simulink model "Backstepping_Quadrator_Attitude"  (R2018a)
settings: Solver=ode4  StartTime=0.0  StopTime=12  FixedStep=1e-4  MaxStep=1e-3  MinStep=1e-4  RelTol=1e-3
libraries: simulink x8, powerlib_meascontrol x1
settings Model: Creator=oussa  LastModifiedBy=oussa

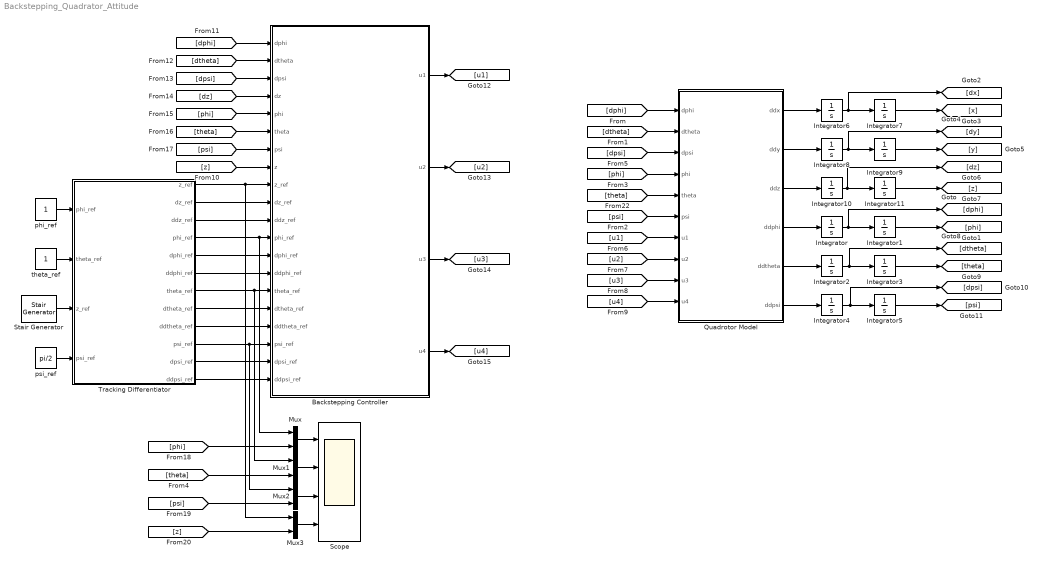
== system Backstepping_Quadrator_Attitude ==
  Backstepping Controller : MATLAB Function  TreatAsAtomicUnit=on
  Integrator : Integrator  InitialCondition=0.001
  Integrator{1..11} (11 alike) : Integrator
  Mux{,1..3} (4 alike) : Mux  Inputs=2
  Quadrotor Model : MATLAB Function  TreatAsAtomicUnit=on
  Scope : Scope  NumInputPorts=4
  Stair Generator : powerlib_meascontrol/Pulse & Signal Generators/Stair Generator  t=[0, 1,3, 5, 8.5,10,12]  e=[0,5,2,9,15,0,0]  Ts=0
      settings: SourceProductName=Simscape Power Systems
  Tracking Differentiator : Subsystem
  phi_ref : Constant
  psi_ref : Constant  Value=pi/2
  theta_ref : Constant
  wires:
  Quadrotor Model/4(ddphi) -> Integrator/1
  Quadrotor Model/5(ddtheta) -> Integrator2/1
  Quadrotor Model/6(ddpsi) -> Integrator4/1
  Integrator10/1 -> [dz], Integrator11/1
  Integrator8/1 -> [dy], Integrator9/1
  Quadrotor Model/1(ddx) -> Integrator6/1
  Quadrotor Model/3(ddz) -> Integrator10/1
  Quadrotor Model/2(ddy) -> Integrator8/1
  Integrator4/1 -> [dpsi], Integrator5/1
  Integrator2/1 -> Integrator3/1, [dtheta]
  Integrator/1 -> Integrator1/1, [dphi]
  Integrator1/1 -> [phi]
  Integrator7/1 -> [x]
  Integrator6/1 -> [dx], Integrator7/1
  Integrator9/1 -> [y]
  Integrator11/1 -> [z]
  Integrator3/1 -> [theta]
  Integrator5/1 -> [psi]
  [dphi] -> Quadrotor Model/1(dphi)
  [dtheta] -> Quadrotor Model/2(dtheta)
  [phi] -> Quadrotor Model/4(phi)
  [theta] -> Quadrotor Model/5(theta)
  [dpsi] -> Quadrotor Model/3(dpsi)
  [psi] -> Quadrotor Model/6(psi)
  [u1] -> Quadrotor Model/7(u1)
  [u2] -> Quadrotor Model/8(u2)
  [u3] -> Quadrotor Model/9(u3)
  [u4] -> Quadrotor Model/10(u4)
  Mux/1 -> Scope/1
  Mux1/1 -> Scope/2
  [psi] -> Mux2/2
  [z] -> Mux3/2
  Mux2/1 -> Scope/3
  Mux3/1 -> Scope/4
  Backstepping Controller/2(u2) -> [u2]
  [z] -> Backstepping Controller/8(z)
  [psi] -> Backstepping Controller/7(psi)
  [theta] -> Backstepping Controller/6(theta)
  [phi] -> Backstepping Controller/5(phi)
  Backstepping Controller/3(u3) -> [u3]
  Backstepping Controller/4(u4) -> [u4]
  [dphi] -> Backstepping Controller/1(dphi)
  [dtheta] -> Backstepping Controller/2(dtheta)
  [dz] -> Backstepping Controller/4(dz)
  [dpsi] -> Backstepping Controller/3(dpsi)
  Tracking Differentiator/1("z_ref ") -> Mux3/1, Backstepping Controller/9(z_ref)
  Tracking Differentiator/2(dz_ref) -> Backstepping Controller/10(dz_ref)
  Tracking Differentiator/3(ddz_ref) -> Backstepping Controller/11(ddz_ref)
  Tracking Differentiator/4("phi_ref ") -> Mux/1, Backstepping Controller/12(phi_ref)
  Tracking Differentiator/5(dphi_ref) -> Backstepping Controller/13(dphi_ref)
  Tracking Differentiator/6(ddphi_ref) -> Backstepping Controller/14(ddphi_ref)
  Tracking Differentiator/7("theta_ref ") -> Mux1/1, Backstepping Controller/15(theta_ref)
  Tracking Differentiator/8("dtheta_ref ") -> Backstepping Controller/16(dtheta_ref)
  Tracking Differentiator/9(ddtheta_ref) -> Backstepping Controller/17(ddtheta_ref)
  Tracking Differentiator/11(dpsi_ref) -> Backstepping Controller/19(dpsi_ref)
  Tracking Differentiator/12(ddpsi_ref) -> Backstepping Controller/20(ddpsi_ref)
  phi_ref/1 -> Tracking Differentiator/1(phi_ref)
  theta_ref/1 -> Tracking Differentiator/2(theta_ref)
  [theta] -> Mux1/2
  [phi] -> Mux/2
  Tracking Differentiator/10("psi_ref ") -> Mux2/1, Backstepping Controller/18(psi_ref)
  psi_ref/1 -> Tracking Differentiator/4(psi_ref)
  Stair Generator/1 -> Tracking Differentiator/3(z_ref)
  Backstepping Controller/1(u1) -> [u1]

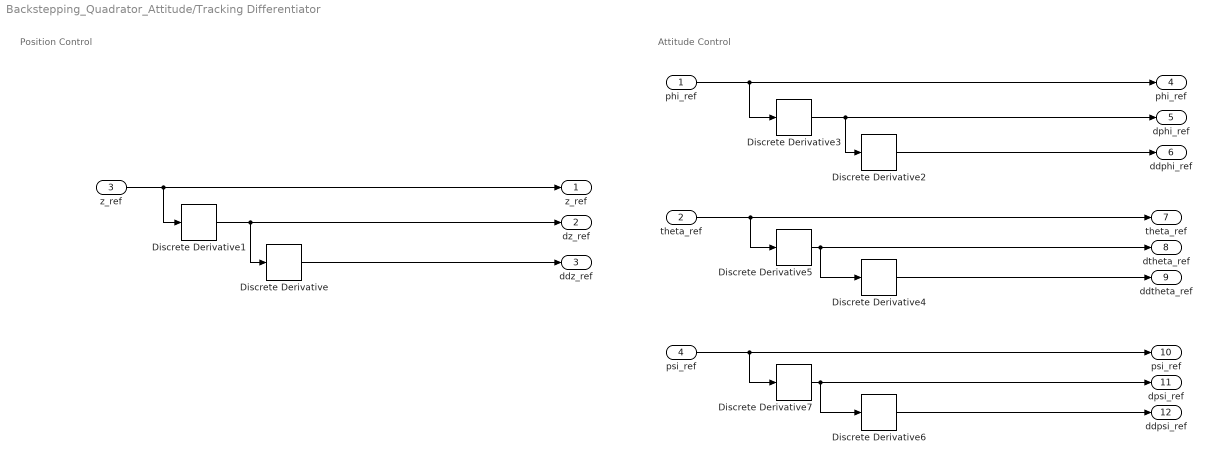
== system Backstepping_Quadrator_Attitude/Tracking Differentiator ==
  note: Attitude Control
  note: Position Control
  phi_ref : Inport
  theta_ref : Inport  Port=2
  z_ref : Inport  Port=3
  psi_ref : Inport  Port=4
  Discrete Derivative{,1..7} (8 alike) : simulink/Discrete/Discrete Derivative  gainval=eps  ICPrevScaledInput=0.0  OutMin=[]  OutMax=[]  OutDataType=fixdt(1, 16)  OutScaling=2^-10  DoSatur=off
  "z_ref " : Outport
  dz_ref : Outport  Port=2
  ddz_ref : Outport  Port=3
  "phi_ref " : Outport  Port=4
  dphi_ref : Outport  Port=5
  ddphi_ref : Outport  Port=6
  "theta_ref " : Outport  Port=7
  "dtheta_ref " : Outport  Port=8
  ddtheta_ref : Outport  Port=9
  "psi_ref " : Outport  Port=10
  dpsi_ref : Outport  Port=11
  ddpsi_ref : Outport  Port=12
  wires:
  Discrete Derivative/1 -> ddz_ref/1
  Discrete Derivative4/1 -> ddtheta_ref/1
  Discrete Derivative1/1 -> Discrete Derivative/1, dz_ref/1
  Discrete Derivative3/1 -> dphi_ref/1, Discrete Derivative2/1
  Discrete Derivative5/1 -> "dtheta_ref "/1, Discrete Derivative4/1
  phi_ref/1 -> "phi_ref "/1, Discrete Derivative3/1
  Discrete Derivative2/1 -> ddphi_ref/1
  theta_ref/1 -> Discrete Derivative5/1, "theta_ref "/1
  psi_ref/1 -> Discrete Derivative7/1, "psi_ref "/1
  Discrete Derivative7/1 -> dpsi_ref/1, Discrete Derivative6/1
  Discrete Derivative6/1 -> ddpsi_ref/1
  z_ref/1 -> Discrete Derivative1/1, "z_ref "/1

== matlab function Backstepping_Quadrator_Attitude/Backstepping Controller ==
  data: dphi input; dtheta input; dpsi input; dz input; phi input; theta input; psi input; z input; z_ref input; dz_ref input; ddz_ref input; phi_ref input; dphi_ref input; ddphi_ref input; theta_ref input; dtheta_ref input; u1 output; u2 output; u3 output; u4 output; ddtheta_ref input; psi_ref input; dpsi_ref input; ddpsi_ref input
function [u1,u2,u3,u4] = Backstepping_Controller(dphi,dtheta,dpsi,dz,phi,theta,psi,z,z_ref,dz_ref,ddz_ref,phi_ref,dphi_ref,ddphi_ref,theta_ref,dtheta_ref,ddtheta_ref,psi_ref,dpsi_ref,ddpsi_ref)
m = 2;
Ix = 1.25;
Iy = 1.25;
Iz = 2.2;
Ir = 1;
g = 9.8;
w = 10;

a1 = (Iy-Iz)/Ix; a2 = -Ir/Ix*w; b1 = 1/Ix;
a3 = (Iz-Ix)/Iy; a4 = Ir/Iy*w; b2 = 1/Iy;
a5= (Ix-Iy)/Iz; b3 = 1/Iz;

k1 = 20;
k2 = k1;
k3 = k1;
k4 = k1;
k5 = k1;
k6 = k1;
k7 = k1;
k8 = k1;

e1 = phi_ref-phi;
e2 = dphi-k1*e1-dphi_ref;
u2 = 1/b1*(-k2*e2+e1+ddphi_ref-k1*(e2+k1*e1)-a1*dtheta*dpsi-a2*dtheta*w);

e3 = theta_ref-theta;
e4 = dtheta-dtheta_ref-k3*e3;
u3 = 1/b2*(-k4*e4+e3-a3*dphi*dpsi-a4*w*dphi+ddtheta_ref-k3*(e4+k3*e3));

e5 = psi_ref-psi;
e6 = dpsi-dpsi_ref-k5*e5;
u4 = 1/b3*(-k6*e6+e5-a5*dphi*dtheta+ddpsi_ref-k5*(e6+k5*e5));

e7 = z_ref-z;
e8 = dz-dz_ref-k7*e7;
u1 = m/(cos(phi)*cos(theta))*(-k8*e8+e7+g-k7*(e8+k7*e7)+ddz_ref);

end

== matlab function Backstepping_Quadrator_Attitude/Quadrotor Model ==
  data: ddx output size=1; dphi input size=1; dtheta input size=1; dpsi input size=1; phi input size=1; theta input size=1; psi input size=1; u1 input size=1; u2 input size=1; u3 input size=1; u4 input size=1; ddy output size=1; ddz output size=1; ddphi output size=1; ddtheta output size=1; ddpsi output size=1
function [ddx,ddy,ddz,ddphi,ddtheta,ddpsi] = Quadrotor(dphi,dtheta,dpsi,phi,theta,psi,u1,u2,u3,u4)
m = 2;
Ix = 1.25;
Iy = 1.25;
Iz = 2.2;
Ir = 1;
g = 9.8;
w = 10;
a1 = (Iy-Iz)/Ix; a2 = -Ir/Ix*w; a3 = 1/Ix;
b1 = (Iz-Ix)/Iy; b2 = Ir/Iy*w; b3 = 1/Iy;
c1= (Ix-Iy)/Iz; c2 = 1/Iz;

ddx = (cos(phi)*sin(theta)*cos(psi)+sin(phi)*sin(psi))*u1/m;
ddy = (cos(phi)*sin(theta)*sin(psi)-sin(phi)*cos(psi))*u1/m;
ddz = -g+(cos(theta)*cos(phi))*u1/m;


ddphi = a1*dtheta*dpsi+a2*w*dtheta+a3*u2;
ddtheta = b1*dpsi*dphi+b2*dphi+b3*u3;
ddpsi = c1*dtheta*dphi+c2*u4;

end
